simulink model "ACT_Lab2_sim"  (R2018b)
settings: Solver=VariableStepAuto  StartTime=0.0  StopTime=10.0  RelTol=1e-3
libraries: simulink x1
settings Model: Creator=gaura  LastModifiedBy=gaura

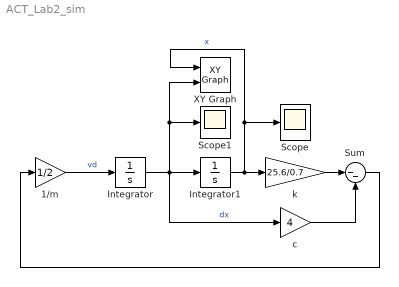
== system ACT_Lab2_sim ==
  "1/m " : Gain  Gain=1/2
  Integrator : Integrator  InitialCondition=0.6
  Integrator1 : Integrator
  Scope : Scope
  Scope1 : Scope
  Sum : Sum  Inputs=|--
  XY Graph : simulink/Sinks/XY Graph  xmin=-0.2  xmax=0.2  ymin=-0.6  ymax=0.6  st=0.01
  "c " : Gain  Gain=4
  "k " : Gain  Gain=25.6/0.7
  wires:
  "1/m "/1 -> Integrator/1  "vd"
  Integrator/1 -> XY Graph/2, Scope1/1, Integrator1/1, "c "/1  "dx"
  Integrator1/1 -> Scope/1, XY Graph/1, "k "/1  "x"
  Sum/1 -> "1/m "/1
  "c "/1 -> Sum/2
  "k "/1 -> Sum/1
